simulink model "c00012M_harness"  (R2018a)
settings: Solver=FixedStepAuto  StartTime=0.0  StopTime=300  FixedStep=0.1  RelTol=1e-3
undefined symbols (not defined in the file): A1, hmax, PriorityTank, R1, R2, sigbuilder_block
(part 3 of 19)

== system c00012M_harness/Eval71 ==
  In1 : Inport
  In2 : Inport  Port=2
  Constant3 : Constant
  Data Type Conversion : DataTypeConversion
  Data Type Conversion1 : DataTypeConversion
  Memory1 : Memory  InitialCondition=1
  Memory2 : Memory  InitialCondition=1
  MinMax : MinMax  Inputs=3
  MinMax1 : MinMax  Inputs=2
  MinMax2 : MinMax  Inputs=2
  ROOut1 : RelationalOperator  Operator===  OutDataTypeStr=boolean  RndMeth=Simplest
  ROOut2 : RelationalOperator  Operator===  OutDataTypeStr=boolean  RndMeth=Simplest
  Out1 : Outport
  wires:
  Data Type Conversion1/1 -> MinMax2/1
  Data Type Conversion/1 -> MinMax1/1
  MinMax1/1 -> Memory1/1, MinMax/1
  MinMax2/1 -> MinMax/2, Memory2/1
  ROOut1/1 -> Data Type Conversion/1
  Memory2/1 -> MinMax2/2
  ROOut2/1 -> Data Type Conversion1/1
  Memory1/1 -> MinMax1/2
  [out2] -> ROOut2/2
  In1/1 -> ROOut1/1
  In2/1 -> ROOut2/1
  [out1] -> ROOut1/2
  MinMax/1 -> Out1/1
  Constant3/1 -> MinMax/3

== system c00012M_harness/Eval72 ==
  In1 : Inport
  In2 : Inport  Port=2
  Constant3 : Constant
  Data Type Conversion : DataTypeConversion
  Data Type Conversion1 : DataTypeConversion
  Memory1 : Memory  InitialCondition=1
  Memory2 : Memory  InitialCondition=1
  MinMax : MinMax  Inputs=3
  MinMax1 : MinMax  Inputs=2
  MinMax2 : MinMax  Inputs=2
  ROOut1 : RelationalOperator  Operator===  OutDataTypeStr=boolean  RndMeth=Simplest
  ROOut2 : RelationalOperator  Operator===  OutDataTypeStr=boolean  RndMeth=Simplest
  Out1 : Outport
  wires:
  Data Type Conversion1/1 -> MinMax2/1
  Data Type Conversion/1 -> MinMax1/1
  MinMax1/1 -> Memory1/1, MinMax/1
  MinMax2/1 -> MinMax/2, Memory2/1
  ROOut1/1 -> Data Type Conversion/1
  Memory2/1 -> MinMax2/2
  ROOut2/1 -> Data Type Conversion1/1
  Memory1/1 -> MinMax1/2
  [out2] -> ROOut2/2
  In1/1 -> ROOut1/1
  In2/1 -> ROOut2/1
  [out1] -> ROOut1/2
  MinMax/1 -> Out1/1
  Constant3/1 -> MinMax/3

== system c00012M_harness/Eval73 ==
  In1 : Inport
  In2 : Inport  Port=2
  Constant3 : Constant
  Data Type Conversion : DataTypeConversion
  Data Type Conversion1 : DataTypeConversion
  Memory1 : Memory  InitialCondition=1
  Memory2 : Memory  InitialCondition=1
  MinMax : MinMax  Inputs=3
  MinMax1 : MinMax  Inputs=2
  MinMax2 : MinMax  Inputs=2
  ROOut1 : RelationalOperator  Operator===  OutDataTypeStr=boolean  RndMeth=Simplest
  ROOut2 : RelationalOperator  Operator===  OutDataTypeStr=boolean  RndMeth=Simplest
  Out1 : Outport
  wires:
  Data Type Conversion1/1 -> MinMax2/1
  Data Type Conversion/1 -> MinMax1/1
  MinMax1/1 -> Memory1/1, MinMax/1
  MinMax2/1 -> MinMax/2, Memory2/1
  ROOut1/1 -> Data Type Conversion/1
  Memory2/1 -> MinMax2/2
  ROOut2/1 -> Data Type Conversion1/1
  Memory1/1 -> MinMax1/2
  [out2] -> ROOut2/2
  In1/1 -> ROOut1/1
  In2/1 -> ROOut2/1
  [out1] -> ROOut1/2
  MinMax/1 -> Out1/1
  Constant3/1 -> MinMax/3

== system c00012M_harness/Eval74 ==
  In1 : Inport
  In2 : Inport  Port=2
  Constant3 : Constant
  Data Type Conversion : DataTypeConversion
  Data Type Conversion1 : DataTypeConversion
  Memory1 : Memory  InitialCondition=1
  Memory2 : Memory  InitialCondition=1
  MinMax : MinMax  Inputs=3
  MinMax1 : MinMax  Inputs=2
  MinMax2 : MinMax  Inputs=2
  ROOut1 : RelationalOperator  Operator===  OutDataTypeStr=boolean  RndMeth=Simplest
  ROOut2 : RelationalOperator  Operator===  OutDataTypeStr=boolean  RndMeth=Simplest
  Out1 : Outport
  wires:
  Data Type Conversion1/1 -> MinMax2/1
  Data Type Conversion/1 -> MinMax1/1
  MinMax1/1 -> Memory1/1, MinMax/1
  MinMax2/1 -> MinMax/2, Memory2/1
  ROOut1/1 -> Data Type Conversion/1
  Memory2/1 -> MinMax2/2
  ROOut2/1 -> Data Type Conversion1/1
  Memory1/1 -> MinMax1/2
  [out2] -> ROOut2/2
  In1/1 -> ROOut1/1
  In2/1 -> ROOut2/1
  [out1] -> ROOut1/2
  MinMax/1 -> Out1/1
  Constant3/1 -> MinMax/3

== system c00012M_harness/Eval75 ==
  In1 : Inport
  In2 : Inport  Port=2
  Constant3 : Constant
  Data Type Conversion : DataTypeConversion
  Data Type Conversion1 : DataTypeConversion
  Memory1 : Memory  InitialCondition=1
  Memory2 : Memory  InitialCondition=1
  MinMax : MinMax  Inputs=3
  MinMax1 : MinMax  Inputs=2
  MinMax2 : MinMax  Inputs=2
  ROOut1 : RelationalOperator  Operator===  OutDataTypeStr=boolean  RndMeth=Simplest
  ROOut2 : RelationalOperator  Operator===  OutDataTypeStr=boolean  RndMeth=Simplest
  Out1 : Outport
  wires:
  Data Type Conversion1/1 -> MinMax2/1
  Data Type Conversion/1 -> MinMax1/1
  MinMax1/1 -> Memory1/1, MinMax/1
  MinMax2/1 -> MinMax/2, Memory2/1
  ROOut1/1 -> Data Type Conversion/1
  Memory2/1 -> MinMax2/2
  ROOut2/1 -> Data Type Conversion1/1
  Memory1/1 -> MinMax1/2
  [out2] -> ROOut2/2
  In1/1 -> ROOut1/1
  In2/1 -> ROOut2/1
  [out1] -> ROOut1/2
  MinMax/1 -> Out1/1
  Constant3/1 -> MinMax/3

== system c00012M_harness/Eval76 ==
  In1 : Inport
  In2 : Inport  Port=2
  Constant3 : Constant
  Data Type Conversion : DataTypeConversion
  Data Type Conversion1 : DataTypeConversion
  Memory1 : Memory  InitialCondition=1
  Memory2 : Memory  InitialCondition=1
  MinMax : MinMax  Inputs=3
  MinMax1 : MinMax  Inputs=2
  MinMax2 : MinMax  Inputs=2
  ROOut1 : RelationalOperator  Operator===  OutDataTypeStr=boolean  RndMeth=Simplest
  ROOut2 : RelationalOperator  Operator===  OutDataTypeStr=boolean  RndMeth=Simplest
  Out1 : Outport
  wires:
  Data Type Conversion1/1 -> MinMax2/1
  Data Type Conversion/1 -> MinMax1/1
  MinMax1/1 -> Memory1/1, MinMax/1
  MinMax2/1 -> MinMax/2, Memory2/1
  ROOut1/1 -> Data Type Conversion/1
  Memory2/1 -> MinMax2/2
  ROOut2/1 -> Data Type Conversion1/1
  Memory1/1 -> MinMax1/2
  [out2] -> ROOut2/2
  In1/1 -> ROOut1/1
  In2/1 -> ROOut2/1
  [out1] -> ROOut1/2
  MinMax/1 -> Out1/1
  Constant3/1 -> MinMax/3

== system c00012M_harness/Eval77 ==
  In1 : Inport
  In2 : Inport  Port=2
  Constant3 : Constant
  Data Type Conversion : DataTypeConversion
  Data Type Conversion1 : DataTypeConversion
  Memory1 : Memory  InitialCondition=1
  Memory2 : Memory  InitialCondition=1
  MinMax : MinMax  Inputs=3
  MinMax1 : MinMax  Inputs=2
  MinMax2 : MinMax  Inputs=2
  ROOut1 : RelationalOperator  Operator===  OutDataTypeStr=boolean  RndMeth=Simplest
  ROOut2 : RelationalOperator  Operator===  OutDataTypeStr=boolean  RndMeth=Simplest
  Out1 : Outport
  wires:
  Data Type Conversion1/1 -> MinMax2/1
  Data Type Conversion/1 -> MinMax1/1
  MinMax1/1 -> Memory1/1, MinMax/1
  MinMax2/1 -> MinMax/2, Memory2/1
  ROOut1/1 -> Data Type Conversion/1
  Memory2/1 -> MinMax2/2
  ROOut2/1 -> Data Type Conversion1/1
  Memory1/1 -> MinMax1/2
  [out2] -> ROOut2/2
  In1/1 -> ROOut1/1
  In2/1 -> ROOut2/1
  [out1] -> ROOut1/2
  MinMax/1 -> Out1/1
  Constant3/1 -> MinMax/3

== system c00012M_harness/Eval78 ==
  In1 : Inport
  In2 : Inport  Port=2
  Constant3 : Constant
  Data Type Conversion : DataTypeConversion
  Data Type Conversion1 : DataTypeConversion
  Memory1 : Memory  InitialCondition=1
  Memory2 : Memory  InitialCondition=1
  MinMax : MinMax  Inputs=3
  MinMax1 : MinMax  Inputs=2
  MinMax2 : MinMax  Inputs=2
  ROOut1 : RelationalOperator  Operator===  OutDataTypeStr=boolean  RndMeth=Simplest
  ROOut2 : RelationalOperator  Operator===  OutDataTypeStr=boolean  RndMeth=Simplest
  Out1 : Outport
  wires:
  Data Type Conversion1/1 -> MinMax2/1
  Data Type Conversion/1 -> MinMax1/1
  MinMax1/1 -> Memory1/1, MinMax/1
  MinMax2/1 -> MinMax/2, Memory2/1
  ROOut1/1 -> Data Type Conversion/1
  Memory2/1 -> MinMax2/2
  ROOut2/1 -> Data Type Conversion1/1
  Memory1/1 -> MinMax1/2
  [out2] -> ROOut2/2
  In1/1 -> ROOut1/1
  In2/1 -> ROOut2/1
  [out1] -> ROOut1/2
  MinMax/1 -> Out1/1
  Constant3/1 -> MinMax/3

== system c00012M_harness/Eval79 ==
  In1 : Inport
  In2 : Inport  Port=2
  Constant3 : Constant
  Data Type Conversion : DataTypeConversion
  Data Type Conversion1 : DataTypeConversion
  Memory1 : Memory  InitialCondition=1
  Memory2 : Memory  InitialCondition=1
  MinMax : MinMax  Inputs=3
  MinMax1 : MinMax  Inputs=2
  MinMax2 : MinMax  Inputs=2
  ROOut1 : RelationalOperator  Operator===  OutDataTypeStr=boolean  RndMeth=Simplest
  ROOut2 : RelationalOperator  Operator===  OutDataTypeStr=boolean  RndMeth=Simplest
  Out1 : Outport
  wires:
  Data Type Conversion1/1 -> MinMax2/1
  Data Type Conversion/1 -> MinMax1/1
  MinMax1/1 -> Memory1/1, MinMax/1
  MinMax2/1 -> MinMax/2, Memory2/1
  ROOut1/1 -> Data Type Conversion/1
  Memory2/1 -> MinMax2/2
  ROOut2/1 -> Data Type Conversion1/1
  Memory1/1 -> MinMax1/2
  [out2] -> ROOut2/2
  In1/1 -> ROOut1/1
  In2/1 -> ROOut2/1
  [out1] -> ROOut1/2
  MinMax/1 -> Out1/1
  Constant3/1 -> MinMax/3

== system c00012M_harness/Eval80 ==
  In1 : Inport
  In2 : Inport  Port=2
  Constant3 : Constant
  Data Type Conversion : DataTypeConversion
  Data Type Conversion1 : DataTypeConversion
  Memory1 : Memory  InitialCondition=1
  Memory2 : Memory  InitialCondition=1
  MinMax : MinMax  Inputs=3
  MinMax1 : MinMax  Inputs=2
  MinMax2 : MinMax  Inputs=2
  ROOut1 : RelationalOperator  Operator===  OutDataTypeStr=boolean  RndMeth=Simplest
  ROOut2 : RelationalOperator  Operator===  OutDataTypeStr=boolean  RndMeth=Simplest
  Out1 : Outport
  wires:
  Data Type Conversion1/1 -> MinMax2/1
  Data Type Conversion/1 -> MinMax1/1
  MinMax1/1 -> Memory1/1, MinMax/1
  MinMax2/1 -> MinMax/2, Memory2/1
  ROOut1/1 -> Data Type Conversion/1
  Memory2/1 -> MinMax2/2
  ROOut2/1 -> Data Type Conversion1/1
  Memory1/1 -> MinMax1/2
  [out2] -> ROOut2/2
  In1/1 -> ROOut1/1
  In2/1 -> ROOut2/1
  [out1] -> ROOut1/2
  MinMax/1 -> Out1/1
  Constant3/1 -> MinMax/3

== system c00012M_harness/Eval81 ==
  In1 : Inport
  In2 : Inport  Port=2
  Constant3 : Constant
  Data Type Conversion : DataTypeConversion
  Data Type Conversion1 : DataTypeConversion
  Memory1 : Memory  InitialCondition=1
  Memory2 : Memory  InitialCondition=1
  MinMax : MinMax  Inputs=3
  MinMax1 : MinMax  Inputs=2
  MinMax2 : MinMax  Inputs=2
  ROOut1 : RelationalOperator  Operator===  OutDataTypeStr=boolean  RndMeth=Simplest
  ROOut2 : RelationalOperator  Operator===  OutDataTypeStr=boolean  RndMeth=Simplest
  Out1 : Outport
  wires:
  Data Type Conversion1/1 -> MinMax2/1
  Data Type Conversion/1 -> MinMax1/1
  MinMax1/1 -> Memory1/1, MinMax/1
  MinMax2/1 -> MinMax/2, Memory2/1
  ROOut1/1 -> Data Type Conversion/1
  Memory2/1 -> MinMax2/2
  ROOut2/1 -> Data Type Conversion1/1
  Memory1/1 -> MinMax1/2
  [out2] -> ROOut2/2
  In1/1 -> ROOut1/1
  In2/1 -> ROOut2/1
  [out1] -> ROOut1/2
  MinMax/1 -> Out1/1
  Constant3/1 -> MinMax/3

== system c00012M_harness/Eval82 ==
  In1 : Inport
  In2 : Inport  Port=2
  Constant3 : Constant
  Data Type Conversion : DataTypeConversion
  Data Type Conversion1 : DataTypeConversion
  Memory1 : Memory  InitialCondition=1
  Memory2 : Memory  InitialCondition=1
  MinMax : MinMax  Inputs=3
  MinMax1 : MinMax  Inputs=2
  MinMax2 : MinMax  Inputs=2
  ROOut1 : RelationalOperator  Operator===  OutDataTypeStr=boolean  RndMeth=Simplest
  ROOut2 : RelationalOperator  Operator===  OutDataTypeStr=boolean  RndMeth=Simplest
  Out1 : Outport
  wires:
  Data Type Conversion1/1 -> MinMax2/1
  Data Type Conversion/1 -> MinMax1/1
  MinMax1/1 -> Memory1/1, MinMax/1
  MinMax2/1 -> MinMax/2, Memory2/1
  ROOut1/1 -> Data Type Conversion/1
  Memory2/1 -> MinMax2/2
  ROOut2/1 -> Data Type Conversion1/1
  Memory1/1 -> MinMax1/2
  [out2] -> ROOut2/2
  In1/1 -> ROOut1/1
  In2/1 -> ROOut2/1
  [out1] -> ROOut1/2
  MinMax/1 -> Out1/1
  Constant3/1 -> MinMax/3

== system c00012M_harness/Inputs ==
  Demux : Demux  Tag=STV Demux  Outputs=10
  FromWs : FromWorkspace  Tag=STV FromWs  VariableName=tuvar  SampleTime=0
  CT1 : Outport  Tag=STV Outport
  F1 : Outport  Tag=STV Outport  Port=2
  E1 : Outport  Tag=STV Outport  Port=3
  T1 : Outport  Tag=STV Outport  Port=4
  EB1 : Outport  Tag=STV Outport  Port=5
  CT2 : Outport  Tag=STV Outport  Port=6
  F2 : Outport  Tag=STV Outport  Port=7
  E2 : Outport  Tag=STV Outport  Port=8
  T2 : Outport  Tag=STV Outport  Port=9
  EB2 : Outport  Tag=STV Outport  Port=10
  wires:
  Demux/10 -> EB2/1
  Demux/9 -> T2/1
  Demux/8 -> E2/1
  Demux/7 -> F2/1
  Demux/6 -> CT2/1
  Demux/5 -> EB1/1
  Demux/4 -> T1/1
  Demux/3 -> E1/1
  Demux/2 -> F1/1
  Demux/1 -> CT1/1
  FromWs/1 -> Demux/1

== system c00012M_harness/M001 ==
  note: Inputs For Tank1
  note: Inputs For Tank3
  note: NAMES
      | --------------------------------------------
      | CT1 = ControlType Tank 1
      | F1 = Fill Tank 1
      | E1 = Empty Tank 1
      | MR1 = Manual Reference Tank1
      | T1 = Temperature Tank 1
      | EB1 = Emergency Button Tank 1
      | LL1 = Liquid Level 1
  note: Inputs For Tank2
  note: VALUES
      | ---------------------------------
      | ControlType = 1 | 2 | 3
      | FillTank = 0 | 1
      | EmptyTank = 0 | 1
      | ManualReference between 0 and 1
      | Tempreature between 0 and 100
      | EmergencyButton = 0 | 1
      | LiquidLevel between 0 and 1 (hmax)
  CT1 : Inport
  F1 : Inport  Port=2
  E1 : Inport  Port=3
  T1 : Inport  Port=4
  EB1 : Inport  Port=5
  CT2 : Inport  Port=6
  F2 : Inport  Port=7
  E2 : Inport  Port=8
  T2 : Inport  Port=9
  EB2 : Inport  Port=10
  Tank1 : Subsystem
  Tank2 : Subsystem
  LL1 : Outport
  LL2 : Outport  Port=2
  wires:
  CT1/1 -> Tank1/1(CT1)
  T2/1 -> Tank2/4(T2)
  E1/1 -> Tank1/3(E1)
  F1/1 -> Tank1/2(F1)
  E2/1 -> Tank2/3(E2)
  F2/1 -> Tank2/2(F2)
  Tank1/1(LL1) -> LL1/1, Tank2/6(LL1)
  T1/1 -> Tank1/4(T1)
  CT2/1 -> Tank2/1(CT2)
  EB2/1 -> Tank2/5(EB2)
  Tank2/1(LL2) -> LL2/1, Tank1/6(LL2)
  EB1/1 -> Tank1/5(EB1)

== system c00012M_harness/M036 ==
  note: VALUES
      | ---------------------------------
      | ControlType = 1 | 2 | 3
      | FillTank = 0 | 1
      | EmptyTank = 0 | 1
      | ManualReference between 0 and 1
      | Tempreature between 0 and 100
      | EmergencyButton = 0 | 1
      | LiquidLevel between 0 and 1 (hmax)
  note: Inputs For Tank2
  note: NAMES
      | --------------------------------------------
      | CT1 = ControlType Tank 1
      | F1 = Fill Tank 1
      | E1 = Empty Tank 1
      | MR1 = Manual Reference Tank1
      | T1 = Temperature Tank 1
      | EB1 = Emergency Button Tank 1
      | LL1 = Liquid Level 1
  note: Inputs For Tank3
  note: Inputs For Tank1
  CT1 : Inport
  F1 : Inport  Port=2
  E1 : Inport  Port=3
  T1 : Inport  Port=4
  EB1 : Inport  Port=5
  CT2 : Inport  Port=6
  F2 : Inport  Port=7
  E2 : Inport  Port=8
  T2 : Inport  Port=9
  EB2 : Inport  Port=10
  Tank1 : Subsystem
  Tank2 : Subsystem
  LL1 : Outport
  LL2 : Outport  Port=2
  wires:
  EB1/1 -> Tank1/5(EB1)
  Tank2/1(LL2) -> LL2/1, Tank1/6(LL2)
  EB2/1 -> Tank2/5(EB2)
  CT2/1 -> Tank2/1(CT2)
  T1/1 -> Tank1/4(T1)
  Tank1/1(LL1) -> LL1/1, Tank2/6(LL1)
  F2/1 -> Tank2/2(F2)
  E2/1 -> Tank2/3(E2)
  F1/1 -> Tank1/2(F1)
  E1/1 -> Tank1/3(E1)
  T2/1 -> Tank2/4(T2)
  CT1/1 -> Tank1/1(CT1)

== system c00012M_harness/M037 ==
  note: VALUES
      | ---------------------------------
      | ControlType = 1 | 2 | 3
      | FillTank = 0 | 1
      | EmptyTank = 0 | 1
      | ManualReference between 0 and 1
      | Tempreature between 0 and 100
      | EmergencyButton = 0 | 1
      | LiquidLevel between 0 and 1 (hmax)
  note: Inputs For Tank2
  note: NAMES
      | --------------------------------------------
      | CT1 = ControlType Tank 1
      | F1 = Fill Tank 1
      | E1 = Empty Tank 1
      | MR1 = Manual Reference Tank1
      | T1 = Temperature Tank 1
      | EB1 = Emergency Button Tank 1
      | LL1 = Liquid Level 1
  note: Inputs For Tank3
  note: Inputs For Tank1
  CT1 : Inport
  F1 : Inport  Port=2
  E1 : Inport  Port=3
  T1 : Inport  Port=4
  EB1 : Inport  Port=5
  CT2 : Inport  Port=6
  F2 : Inport  Port=7
  E2 : Inport  Port=8
  T2 : Inport  Port=9
  EB2 : Inport  Port=10
  Tank1 : Subsystem
  Tank2 : Subsystem
  LL1 : Outport
  LL2 : Outport  Port=2
  wires:
  EB1/1 -> Tank1/5(EB1)
  Tank2/1(LL2) -> LL2/1, Tank1/6(LL2)
  EB2/1 -> Tank2/5(EB2)
  CT2/1 -> Tank2/1(CT2)
  T1/1 -> Tank1/4(T1)
  Tank1/1(LL1) -> LL1/1, Tank2/6(LL1)
  F2/1 -> Tank2/2(F2)
  E2/1 -> Tank2/3(E2)
  F1/1 -> Tank1/2(F1)
  E1/1 -> Tank1/3(E1)
  T2/1 -> Tank2/4(T2)
  CT1/1 -> Tank1/1(CT1)

== system c00012M_harness/M038 ==
  note: VALUES
      | ---------------------------------
      | ControlType = 1 | 2 | 3
      | FillTank = 0 | 1
      | EmptyTank = 0 | 1
      | ManualReference between 0 and 1
      | Tempreature between 0 and 100
      | EmergencyButton = 0 | 1
      | LiquidLevel between 0 and 1 (hmax)
  note: Inputs For Tank2
  note: NAMES
      | --------------------------------------------
      | CT1 = ControlType Tank 1
      | F1 = Fill Tank 1
      | E1 = Empty Tank 1
      | MR1 = Manual Reference Tank1
      | T1 = Temperature Tank 1
      | EB1 = Emergency Button Tank 1
      | LL1 = Liquid Level 1
  note: Inputs For Tank3
  note: Inputs For Tank1
  CT1 : Inport
  F1 : Inport  Port=2
  E1 : Inport  Port=3
  T1 : Inport  Port=4
  EB1 : Inport  Port=5
  CT2 : Inport  Port=6
  F2 : Inport  Port=7
  E2 : Inport  Port=8
  T2 : Inport  Port=9
  EB2 : Inport  Port=10
  Tank1 : Subsystem
  Tank2 : Subsystem
  LL1 : Outport
  LL2 : Outport  Port=2
  wires:
  EB1/1 -> Tank1/5(EB1)
  Tank2/1(LL2) -> LL2/1, Tank1/6(LL2)
  EB2/1 -> Tank2/5(EB2)
  CT2/1 -> Tank2/1(CT2)
  T1/1 -> Tank1/4(T1)
  Tank1/1(LL1) -> LL1/1, Tank2/6(LL1)
  F2/1 -> Tank2/2(F2)
  E2/1 -> Tank2/3(E2)
  F1/1 -> Tank1/2(F1)
  E1/1 -> Tank1/3(E1)
  T2/1 -> Tank2/4(T2)
  CT1/1 -> Tank1/1(CT1)

== system c00012M_harness/M039 ==
  note: VALUES
      | ---------------------------------
      | ControlType = 1 | 2 | 3
      | FillTank = 0 | 1
      | EmptyTank = 0 | 1
      | ManualReference between 0 and 1
      | Tempreature between 0 and 100
      | EmergencyButton = 0 | 1
      | LiquidLevel between 0 and 1 (hmax)
  note: Inputs For Tank2
  note: NAMES
      | --------------------------------------------
      | CT1 = ControlType Tank 1
      | F1 = Fill Tank 1
      | E1 = Empty Tank 1
      | MR1 = Manual Reference Tank1
      | T1 = Temperature Tank 1
      | EB1 = Emergency Button Tank 1
      | LL1 = Liquid Level 1
  note: Inputs For Tank3
  note: Inputs For Tank1
  CT1 : Inport
  F1 : Inport  Port=2
  E1 : Inport  Port=3
  T1 : Inport  Port=4
  EB1 : Inport  Port=5
  CT2 : Inport  Port=6
  F2 : Inport  Port=7
  E2 : Inport  Port=8
  T2 : Inport  Port=9
  EB2 : Inport  Port=10
  Tank1 : Subsystem
  Tank2 : Subsystem
  LL1 : Outport
  LL2 : Outport  Port=2
  wires:
  EB1/1 -> Tank1/5(EB1)
  Tank2/1(LL2) -> LL2/1, Tank1/6(LL2)
  EB2/1 -> Tank2/5(EB2)
  CT2/1 -> Tank2/1(CT2)
  T1/1 -> Tank1/4(T1)
  Tank1/1(LL1) -> LL1/1, Tank2/6(LL1)
  F2/1 -> Tank2/2(F2)
  E2/1 -> Tank2/3(E2)
  F1/1 -> Tank1/2(F1)
  E1/1 -> Tank1/3(E1)
  T2/1 -> Tank2/4(T2)
  CT1/1 -> Tank1/1(CT1)

== system c00012M_harness/M040 ==
  note: VALUES
      | ---------------------------------
      | ControlType = 1 | 2 | 3
      | FillTank = 0 | 1
      | EmptyTank = 0 | 1
      | ManualReference between 0 and 1
      | Tempreature between 0 and 100
      | EmergencyButton = 0 | 1
      | LiquidLevel between 0 and 1 (hmax)
  note: Inputs For Tank2
  note: NAMES
      | --------------------------------------------
      | CT1 = ControlType Tank 1
      | F1 = Fill Tank 1
      | E1 = Empty Tank 1
      | MR1 = Manual Reference Tank1
      | T1 = Temperature Tank 1
      | EB1 = Emergency Button Tank 1
      | LL1 = Liquid Level 1
  note: Inputs For Tank3
  note: Inputs For Tank1
  CT1 : Inport
  F1 : Inport  Port=2
  E1 : Inport  Port=3
  T1 : Inport  Port=4
  EB1 : Inport  Port=5
  CT2 : Inport  Port=6
  F2 : Inport  Port=7
  E2 : Inport  Port=8
  T2 : Inport  Port=9
  EB2 : Inport  Port=10
  Tank1 : Subsystem
  Tank2 : Subsystem
  LL1 : Outport
  LL2 : Outport  Port=2
  wires:
  EB1/1 -> Tank1/5(EB1)
  Tank2/1(LL2) -> LL2/1, Tank1/6(LL2)
  EB2/1 -> Tank2/5(EB2)
  CT2/1 -> Tank2/1(CT2)
  T1/1 -> Tank1/4(T1)
  Tank1/1(LL1) -> LL1/1, Tank2/6(LL1)
  F2/1 -> Tank2/2(F2)
  E2/1 -> Tank2/3(E2)
  F1/1 -> Tank1/2(F1)
  E1/1 -> Tank1/3(E1)
  T2/1 -> Tank2/4(T2)
  CT1/1 -> Tank1/1(CT1)

== system c00012M_harness/M041 ==
  note: VALUES
      | ---------------------------------
      | ControlType = 1 | 2 | 3
      | FillTank = 0 | 1
      | EmptyTank = 0 | 1
      | ManualReference between 0 and 1
      | Tempreature between 0 and 100
      | EmergencyButton = 0 | 1
      | LiquidLevel between 0 and 1 (hmax)
  note: Inputs For Tank2
  note: NAMES
      | --------------------------------------------
      | CT1 = ControlType Tank 1
      | F1 = Fill Tank 1
      | E1 = Empty Tank 1
      | MR1 = Manual Reference Tank1
      | T1 = Temperature Tank 1
      | EB1 = Emergency Button Tank 1
      | LL1 = Liquid Level 1
  note: Inputs For Tank3
  note: Inputs For Tank1
  CT1 : Inport
  F1 : Inport  Port=2
  E1 : Inport  Port=3
  T1 : Inport  Port=4
  EB1 : Inport  Port=5
  CT2 : Inport  Port=6
  F2 : Inport  Port=7
  E2 : Inport  Port=8
  T2 : Inport  Port=9
  EB2 : Inport  Port=10
  Tank1 : Subsystem
  Tank2 : Subsystem
  LL1 : Outport
  LL2 : Outport  Port=2
  wires:
  EB1/1 -> Tank1/5(EB1)
  Tank2/1(LL2) -> LL2/1, Tank1/6(LL2)
  EB2/1 -> Tank2/5(EB2)
  CT2/1 -> Tank2/1(CT2)
  T1/1 -> Tank1/4(T1)
  Tank1/1(LL1) -> LL1/1, Tank2/6(LL1)
  F2/1 -> Tank2/2(F2)
  E2/1 -> Tank2/3(E2)
  F1/1 -> Tank1/2(F1)
  E1/1 -> Tank1/3(E1)
  T2/1 -> Tank2/4(T2)
  CT1/1 -> Tank1/1(CT1)

== system c00012M_harness/M042 ==
  note: VALUES
      | ---------------------------------
      | ControlType = 1 | 2 | 3
      | FillTank = 0 | 1
      | EmptyTank = 0 | 1
      | ManualReference between 0 and 1
      | Tempreature between 0 and 100
      | EmergencyButton = 0 | 1
      | LiquidLevel between 0 and 1 (hmax)
  note: Inputs For Tank2
  note: NAMES
      | --------------------------------------------
      | CT1 = ControlType Tank 1
      | F1 = Fill Tank 1
      | E1 = Empty Tank 1
      | MR1 = Manual Reference Tank1
      | T1 = Temperature Tank 1
      | EB1 = Emergency Button Tank 1
      | LL1 = Liquid Level 1
  note: Inputs For Tank3
  note: Inputs For Tank1
  CT1 : Inport
  F1 : Inport  Port=2
  E1 : Inport  Port=3
  T1 : Inport  Port=4
  EB1 : Inport  Port=5
  CT2 : Inport  Port=6
  F2 : Inport  Port=7
  E2 : Inport  Port=8
  T2 : Inport  Port=9
  EB2 : Inport  Port=10
  Tank1 : Subsystem
  Tank2 : Subsystem
  LL1 : Outport
  LL2 : Outport  Port=2
  wires:
  EB1/1 -> Tank1/5(EB1)
  Tank2/1(LL2) -> LL2/1, Tank1/6(LL2)
  EB2/1 -> Tank2/5(EB2)
  CT2/1 -> Tank2/1(CT2)
  T1/1 -> Tank1/4(T1)
  Tank1/1(LL1) -> LL1/1, Tank2/6(LL1)
  F2/1 -> Tank2/2(F2)
  E2/1 -> Tank2/3(E2)
  F1/1 -> Tank1/2(F1)
  E1/1 -> Tank1/3(E1)
  T2/1 -> Tank2/4(T2)
  CT1/1 -> Tank1/1(CT1)

== system c00012M_harness/M043 ==
  note: VALUES
      | ---------------------------------
      | ControlType = 1 | 2 | 3
      | FillTank = 0 | 1
      | EmptyTank = 0 | 1
      | ManualReference between 0 and 1
      | Tempreature between 0 and 100
      | EmergencyButton = 0 | 1
      | LiquidLevel between 0 and 1 (hmax)
  note: Inputs For Tank2
  note: NAMES
      | --------------------------------------------
      | CT1 = ControlType Tank 1
      | F1 = Fill Tank 1
      | E1 = Empty Tank 1
      | MR1 = Manual Reference Tank1
      | T1 = Temperature Tank 1
      | EB1 = Emergency Button Tank 1
      | LL1 = Liquid Level 1
  note: Inputs For Tank3
  note: Inputs For Tank1
  CT1 : Inport
  F1 : Inport  Port=2
  E1 : Inport  Port=3
  T1 : Inport  Port=4
  EB1 : Inport  Port=5
  CT2 : Inport  Port=6
  F2 : Inport  Port=7
  E2 : Inport  Port=8
  T2 : Inport  Port=9
  EB2 : Inport  Port=10
  Tank1 : Subsystem
  Tank2 : Subsystem
  LL1 : Outport
  LL2 : Outport  Port=2
  wires:
  EB1/1 -> Tank1/5(EB1)
  Tank2/1(LL2) -> LL2/1, Tank1/6(LL2)
  EB2/1 -> Tank2/5(EB2)
  CT2/1 -> Tank2/1(CT2)
  T1/1 -> Tank1/4(T1)
  Tank1/1(LL1) -> LL1/1, Tank2/6(LL1)
  F2/1 -> Tank2/2(F2)
  E2/1 -> Tank2/3(E2)
  F1/1 -> Tank1/2(F1)
  E1/1 -> Tank1/3(E1)
  T2/1 -> Tank2/4(T2)
  CT1/1 -> Tank1/1(CT1)

== system c00012M_harness/M044 ==
  note: VALUES
      | ---------------------------------
      | ControlType = 1 | 2 | 3
      | FillTank = 0 | 1
      | EmptyTank = 0 | 1
      | ManualReference between 0 and 1
      | Tempreature between 0 and 100
      | EmergencyButton = 0 | 1
      | LiquidLevel between 0 and 1 (hmax)
  note: Inputs For Tank2
  note: NAMES
      | --------------------------------------------
      | CT1 = ControlType Tank 1
      | F1 = Fill Tank 1
      | E1 = Empty Tank 1
      | MR1 = Manual Reference Tank1
      | T1 = Temperature Tank 1
      | EB1 = Emergency Button Tank 1
      | LL1 = Liquid Level 1
  note: Inputs For Tank3
  note: Inputs For Tank1
  CT1 : Inport
  F1 : Inport  Port=2
  E1 : Inport  Port=3
  T1 : Inport  Port=4
  EB1 : Inport  Port=5
  CT2 : Inport  Port=6
  F2 : Inport  Port=7
  E2 : Inport  Port=8
  T2 : Inport  Port=9
  EB2 : Inport  Port=10
  Tank1 : Subsystem
  Tank2 : Subsystem
  LL1 : Outport
  LL2 : Outport  Port=2
  wires:
  EB1/1 -> Tank1/5(EB1)
  Tank2/1(LL2) -> LL2/1, Tank1/6(LL2)
  EB2/1 -> Tank2/5(EB2)
  CT2/1 -> Tank2/1(CT2)
  T1/1 -> Tank1/4(T1)
  Tank1/1(LL1) -> LL1/1, Tank2/6(LL1)
  F2/1 -> Tank2/2(F2)
  E2/1 -> Tank2/3(E2)
  F1/1 -> Tank1/2(F1)
  E1/1 -> Tank1/3(E1)
  T2/1 -> Tank2/4(T2)
  CT1/1 -> Tank1/1(CT1)

== system c00012M_harness/M045 ==
  note: VALUES
      | ---------------------------------
      | ControlType = 1 | 2 | 3
      | FillTank = 0 | 1
      | EmptyTank = 0 | 1
      | ManualReference between 0 and 1
      | Tempreature between 0 and 100
      | EmergencyButton = 0 | 1
      | LiquidLevel between 0 and 1 (hmax)
  note: Inputs For Tank2
  note: NAMES
      | --------------------------------------------
      | CT1 = ControlType Tank 1
      | F1 = Fill Tank 1
      | E1 = Empty Tank 1
      | MR1 = Manual Reference Tank1
      | T1 = Temperature Tank 1
      | EB1 = Emergency Button Tank 1
      | LL1 = Liquid Level 1
  note: Inputs For Tank3
  note: Inputs For Tank1
  CT1 : Inport
  F1 : Inport  Port=2
  E1 : Inport  Port=3
  T1 : Inport  Port=4
  EB1 : Inport  Port=5
  CT2 : Inport  Port=6
  F2 : Inport  Port=7
  E2 : Inport  Port=8
  T2 : Inport  Port=9
  EB2 : Inport  Port=10
  Tank1 : Subsystem
  Tank2 : Subsystem
  LL1 : Outport
  LL2 : Outport  Port=2
  wires:
  EB1/1 -> Tank1/5(EB1)
  Tank2/1(LL2) -> LL2/1, Tank1/6(LL2)
  EB2/1 -> Tank2/5(EB2)
  CT2/1 -> Tank2/1(CT2)
  T1/1 -> Tank1/4(T1)
  Tank1/1(LL1) -> LL1/1, Tank2/6(LL1)
  F2/1 -> Tank2/2(F2)
  E2/1 -> Tank2/3(E2)
  F1/1 -> Tank1/2(F1)
  E1/1 -> Tank1/3(E1)
  T2/1 -> Tank2/4(T2)
  CT1/1 -> Tank1/1(CT1)

== system c00012M_harness/M058 ==
  note: VALUES
      | ---------------------------------
      | ControlType = 1 | 2 | 3
      | FillTank = 0 | 1
      | EmptyTank = 0 | 1
      | ManualReference between 0 and 1
      | Tempreature between 0 and 100
      | EmergencyButton = 0 | 1
      | LiquidLevel between 0 and 1 (hmax)
  note: Inputs For Tank2
  note: NAMES
      | --------------------------------------------
      | CT1 = ControlType Tank 1
      | F1 = Fill Tank 1
      | E1 = Empty Tank 1
      | MR1 = Manual Reference Tank1
      | T1 = Temperature Tank 1
      | EB1 = Emergency Button Tank 1
      | LL1 = Liquid Level 1
  note: Inputs For Tank3
  note: Inputs For Tank1
  CT1 : Inport
  F1 : Inport  Port=2
  E1 : Inport  Port=3
  T1 : Inport  Port=4
  EB1 : Inport  Port=5
  CT2 : Inport  Port=6
  F2 : Inport  Port=7
  E2 : Inport  Port=8
  T2 : Inport  Port=9
  EB2 : Inport  Port=10
  Tank1 : Subsystem
  Tank2 : Subsystem
  LL1 : Outport
  LL2 : Outport  Port=2
  wires:
  EB1/1 -> Tank1/5(EB1)
  Tank2/1(LL2) -> LL2/1, Tank1/6(LL2)
  EB2/1 -> Tank2/5(EB2)
  CT2/1 -> Tank2/1(CT2)
  T1/1 -> Tank1/4(T1)
  Tank1/1(LL1) -> LL1/1, Tank2/6(LL1)
  F2/1 -> Tank2/2(F2)
  E2/1 -> Tank2/3(E2)
  F1/1 -> Tank1/2(F1)
  E1/1 -> Tank1/3(E1)
  T2/1 -> Tank2/4(T2)
  CT1/1 -> Tank1/1(CT1)

== system c00012M_harness/M059 ==
  note: VALUES
      | ---------------------------------
      | ControlType = 1 | 2 | 3
      | FillTank = 0 | 1
      | EmptyTank = 0 | 1
      | ManualReference between 0 and 1
      | Tempreature between 0 and 100
      | EmergencyButton = 0 | 1
      | LiquidLevel between 0 and 1 (hmax)
  note: Inputs For Tank2
  note: NAMES
      | --------------------------------------------
      | CT1 = ControlType Tank 1
      | F1 = Fill Tank 1
      | E1 = Empty Tank 1
      | MR1 = Manual Reference Tank1
      | T1 = Temperature Tank 1
      | EB1 = Emergency Button Tank 1
      | LL1 = Liquid Level 1
  note: Inputs For Tank3
  note: Inputs For Tank1
  CT1 : Inport
  F1 : Inport  Port=2
  E1 : Inport  Port=3
  T1 : Inport  Port=4
  EB1 : Inport  Port=5
  CT2 : Inport  Port=6
  F2 : Inport  Port=7
  E2 : Inport  Port=8
  T2 : Inport  Port=9
  EB2 : Inport  Port=10
  Tank1 : Subsystem
  Tank2 : Subsystem
  LL1 : Outport
  LL2 : Outport  Port=2
  wires:
  EB1/1 -> Tank1/5(EB1)
  Tank2/1(LL2) -> LL2/1, Tank1/6(LL2)
  EB2/1 -> Tank2/5(EB2)
  CT2/1 -> Tank2/1(CT2)
  T1/1 -> Tank1/4(T1)
  Tank1/1(LL1) -> LL1/1, Tank2/6(LL1)
  F2/1 -> Tank2/2(F2)
  E2/1 -> Tank2/3(E2)
  F1/1 -> Tank1/2(F1)
  E1/1 -> Tank1/3(E1)
  T2/1 -> Tank2/4(T2)
  CT1/1 -> Tank1/1(CT1)

== system c00012M_harness/M060 ==
  note: VALUES
      | ---------------------------------
      | ControlType = 1 | 2 | 3
      | FillTank = 0 | 1
      | EmptyTank = 0 | 1
      | ManualReference between 0 and 1
      | Tempreature between 0 and 100
      | EmergencyButton = 0 | 1
      | LiquidLevel between 0 and 1 (hmax)
  note: Inputs For Tank2
  note: NAMES
      | --------------------------------------------
      | CT1 = ControlType Tank 1
      | F1 = Fill Tank 1
      | E1 = Empty Tank 1
      | MR1 = Manual Reference Tank1
      | T1 = Temperature Tank 1
      | EB1 = Emergency Button Tank 1
      | LL1 = Liquid Level 1
  note: Inputs For Tank3
  note: Inputs For Tank1
  CT1 : Inport
  F1 : Inport  Port=2
  E1 : Inport  Port=3
  T1 : Inport  Port=4
  EB1 : Inport  Port=5
  CT2 : Inport  Port=6
  F2 : Inport  Port=7
  E2 : Inport  Port=8
  T2 : Inport  Port=9
  EB2 : Inport  Port=10
  Tank1 : Subsystem
  Tank2 : Subsystem
  LL1 : Outport
  LL2 : Outport  Port=2
  wires:
  EB1/1 -> Tank1/5(EB1)
  Tank2/1(LL2) -> LL2/1, Tank1/6(LL2)
  EB2/1 -> Tank2/5(EB2)
  CT2/1 -> Tank2/1(CT2)
  T1/1 -> Tank1/4(T1)
  Tank1/1(LL1) -> LL1/1, Tank2/6(LL1)
  F2/1 -> Tank2/2(F2)
  E2/1 -> Tank2/3(E2)
  F1/1 -> Tank1/2(F1)
  E1/1 -> Tank1/3(E1)
  T2/1 -> Tank2/4(T2)
  CT1/1 -> Tank1/1(CT1)

== system c00012M_harness/M061 ==
  note: VALUES
      | ---------------------------------
      | ControlType = 1 | 2 | 3
      | FillTank = 0 | 1
      | EmptyTank = 0 | 1
      | ManualReference between 0 and 1
      | Tempreature between 0 and 100
      | EmergencyButton = 0 | 1
      | LiquidLevel between 0 and 1 (hmax)
  note: Inputs For Tank2
  note: NAMES
      | --------------------------------------------
      | CT1 = ControlType Tank 1
      | F1 = Fill Tank 1
      | E1 = Empty Tank 1
      | MR1 = Manual Reference Tank1
      | T1 = Temperature Tank 1
      | EB1 = Emergency Button Tank 1
      | LL1 = Liquid Level 1
  note: Inputs For Tank3
  note: Inputs For Tank1
  CT1 : Inport
  F1 : Inport  Port=2
  E1 : Inport  Port=3
  T1 : Inport  Port=4
  EB1 : Inport  Port=5
  CT2 : Inport  Port=6
  F2 : Inport  Port=7
  E2 : Inport  Port=8
  T2 : Inport  Port=9
  EB2 : Inport  Port=10
  Tank1 : Subsystem
  Tank2 : Subsystem
  LL1 : Outport
  LL2 : Outport  Port=2
  wires:
  EB1/1 -> Tank1/5(EB1)
  Tank2/1(LL2) -> LL2/1, Tank1/6(LL2)
  EB2/1 -> Tank2/5(EB2)
  CT2/1 -> Tank2/1(CT2)
  T1/1 -> Tank1/4(T1)
  Tank1/1(LL1) -> LL1/1, Tank2/6(LL1)
  F2/1 -> Tank2/2(F2)
  E2/1 -> Tank2/3(E2)
  F1/1 -> Tank1/2(F1)
  E1/1 -> Tank1/3(E1)
  T2/1 -> Tank2/4(T2)
  CT1/1 -> Tank1/1(CT1)

== system c00012M_harness/M062 ==
  note: VALUES
      | ---------------------------------
      | ControlType = 1 | 2 | 3
      | FillTank = 0 | 1
      | EmptyTank = 0 | 1
      | ManualReference between 0 and 1
      | Tempreature between 0 and 100
      | EmergencyButton = 0 | 1
      | LiquidLevel between 0 and 1 (hmax)
  note: Inputs For Tank2
  note: NAMES
      | --------------------------------------------
      | CT1 = ControlType Tank 1
      | F1 = Fill Tank 1
      | E1 = Empty Tank 1
      | MR1 = Manual Reference Tank1
      | T1 = Temperature Tank 1
      | EB1 = Emergency Button Tank 1
      | LL1 = Liquid Level 1
  note: Inputs For Tank3
  note: Inputs For Tank1
  CT1 : Inport
  F1 : Inport  Port=2
  E1 : Inport  Port=3
  T1 : Inport  Port=4
  EB1 : Inport  Port=5
  CT2 : Inport  Port=6
  F2 : Inport  Port=7
  E2 : Inport  Port=8
  T2 : Inport  Port=9
  EB2 : Inport  Port=10
  Tank1 : Subsystem
  Tank2 : Subsystem
  LL1 : Outport
  LL2 : Outport  Port=2
  wires:
  EB1/1 -> Tank1/5(EB1)
  Tank2/1(LL2) -> LL2/1, Tank1/6(LL2)
  EB2/1 -> Tank2/5(EB2)
  CT2/1 -> Tank2/1(CT2)
  T1/1 -> Tank1/4(T1)
  Tank1/1(LL1) -> LL1/1, Tank2/6(LL1)
  F2/1 -> Tank2/2(F2)
  E2/1 -> Tank2/3(E2)
  F1/1 -> Tank1/2(F1)
  E1/1 -> Tank1/3(E1)
  T2/1 -> Tank2/4(T2)
  CT1/1 -> Tank1/1(CT1)

== system c00012M_harness/M063 ==
  note: VALUES
      | ---------------------------------
      | ControlType = 1 | 2 | 3
      | FillTank = 0 | 1
      | EmptyTank = 0 | 1
      | ManualReference between 0 and 1
      | Tempreature between 0 and 100
      | EmergencyButton = 0 | 1
      | LiquidLevel between 0 and 1 (hmax)
  note: Inputs For Tank2
  note: NAMES
      | --------------------------------------------
      | CT1 = ControlType Tank 1
      | F1 = Fill Tank 1
      | E1 = Empty Tank 1
      | MR1 = Manual Reference Tank1
      | T1 = Temperature Tank 1
      | EB1 = Emergency Button Tank 1
      | LL1 = Liquid Level 1
  note: Inputs For Tank3
  note: Inputs For Tank1
  CT1 : Inport
  F1 : Inport  Port=2
  E1 : Inport  Port=3
  T1 : Inport  Port=4
  EB1 : Inport  Port=5
  CT2 : Inport  Port=6
  F2 : Inport  Port=7
  E2 : Inport  Port=8
  T2 : Inport  Port=9
  EB2 : Inport  Port=10
  Tank1 : Subsystem
  Tank2 : Subsystem
  LL1 : Outport
  LL2 : Outport  Port=2
  wires:
  EB1/1 -> Tank1/5(EB1)
  Tank2/1(LL2) -> LL2/1, Tank1/6(LL2)
  EB2/1 -> Tank2/5(EB2)
  CT2/1 -> Tank2/1(CT2)
  T1/1 -> Tank1/4(T1)
  Tank1/1(LL1) -> LL1/1, Tank2/6(LL1)
  F2/1 -> Tank2/2(F2)
  E2/1 -> Tank2/3(E2)
  F1/1 -> Tank1/2(F1)
  E1/1 -> Tank1/3(E1)
  T2/1 -> Tank2/4(T2)
  CT1/1 -> Tank1/1(CT1)

== system c00012M_harness/M064 ==
  note: VALUES
      | ---------------------------------
      | ControlType = 1 | 2 | 3
      | FillTank = 0 | 1
      | EmptyTank = 0 | 1
      | ManualReference between 0 and 1
      | Tempreature between 0 and 100
      | EmergencyButton = 0 | 1
      | LiquidLevel between 0 and 1 (hmax)
  note: Inputs For Tank2
  note: NAMES
      | --------------------------------------------
      | CT1 = ControlType Tank 1
      | F1 = Fill Tank 1
      | E1 = Empty Tank 1
      | MR1 = Manual Reference Tank1
      | T1 = Temperature Tank 1
      | EB1 = Emergency Button Tank 1
      | LL1 = Liquid Level 1
  note: Inputs For Tank3
  note: Inputs For Tank1
  CT1 : Inport
  F1 : Inport  Port=2
  E1 : Inport  Port=3
  T1 : Inport  Port=4
  EB1 : Inport  Port=5
  CT2 : Inport  Port=6
  F2 : Inport  Port=7
  E2 : Inport  Port=8
  T2 : Inport  Port=9
  EB2 : Inport  Port=10
  Tank1 : Subsystem
  Tank2 : Subsystem
  LL1 : Outport
  LL2 : Outport  Port=2
  wires:
  EB1/1 -> Tank1/5(EB1)
  Tank2/1(LL2) -> LL2/1, Tank1/6(LL2)
  EB2/1 -> Tank2/5(EB2)
  CT2/1 -> Tank2/1(CT2)
  T1/1 -> Tank1/4(T1)
  Tank1/1(LL1) -> LL1/1, Tank2/6(LL1)
  F2/1 -> Tank2/2(F2)
  E2/1 -> Tank2/3(E2)
  F1/1 -> Tank1/2(F1)
  E1/1 -> Tank1/3(E1)
  T2/1 -> Tank2/4(T2)
  CT1/1 -> Tank1/1(CT1)

== system c00012M_harness/M065 ==
  note: VALUES
      | ---------------------------------
      | ControlType = 1 | 2 | 3
      | FillTank = 0 | 1
      | EmptyTank = 0 | 1
      | ManualReference between 0 and 1
      | Tempreature between 0 and 100
      | EmergencyButton = 0 | 1
      | LiquidLevel between 0 and 1 (hmax)
  note: Inputs For Tank2
  note: NAMES
      | --------------------------------------------
      | CT1 = ControlType Tank 1
      | F1 = Fill Tank 1
      | E1 = Empty Tank 1
      | MR1 = Manual Reference Tank1
      | T1 = Temperature Tank 1
      | EB1 = Emergency Button Tank 1
      | LL1 = Liquid Level 1
  note: Inputs For Tank3
  note: Inputs For Tank1
  CT1 : Inport
  F1 : Inport  Port=2
  E1 : Inport  Port=3
  T1 : Inport  Port=4
  EB1 : Inport  Port=5
  CT2 : Inport  Port=6
  F2 : Inport  Port=7
  E2 : Inport  Port=8
  T2 : Inport  Port=9
  EB2 : Inport  Port=10
  Tank1 : Subsystem
  Tank2 : Subsystem
  LL1 : Outport
  LL2 : Outport  Port=2
  wires:
  EB1/1 -> Tank1/5(EB1)
  Tank2/1(LL2) -> LL2/1, Tank1/6(LL2)
  EB2/1 -> Tank2/5(EB2)
  CT2/1 -> Tank2/1(CT2)
  T1/1 -> Tank1/4(T1)
  Tank1/1(LL1) -> LL1/1, Tank2/6(LL1)
  F2/1 -> Tank2/2(F2)
  E2/1 -> Tank2/3(E2)
  F1/1 -> Tank1/2(F1)
  E1/1 -> Tank1/3(E1)
  T2/1 -> Tank2/4(T2)
  CT1/1 -> Tank1/1(CT1)

== system c00012M_harness/M066 ==
  note: VALUES
      | ---------------------------------
      | ControlType = 1 | 2 | 3
      | FillTank = 0 | 1
      | EmptyTank = 0 | 1
      | ManualReference between 0 and 1
      | Tempreature between 0 and 100
      | EmergencyButton = 0 | 1
      | LiquidLevel between 0 and 1 (hmax)
  note: Inputs For Tank2
  note: NAMES
      | --------------------------------------------
      | CT1 = ControlType Tank 1
      | F1 = Fill Tank 1
      | E1 = Empty Tank 1
      | MR1 = Manual Reference Tank1
      | T1 = Temperature Tank 1
      | EB1 = Emergency Button Tank 1
      | LL1 = Liquid Level 1
  note: Inputs For Tank3
  note: Inputs For Tank1
  CT1 : Inport
  F1 : Inport  Port=2
  E1 : Inport  Port=3
  T1 : Inport  Port=4
  EB1 : Inport  Port=5
  CT2 : Inport  Port=6
  F2 : Inport  Port=7
  E2 : Inport  Port=8
  T2 : Inport  Port=9
  EB2 : Inport  Port=10
  Tank1 : Subsystem
  Tank2 : Subsystem
  LL1 : Outport
  LL2 : Outport  Port=2
  wires:
  EB1/1 -> Tank1/5(EB1)
  Tank2/1(LL2) -> LL2/1, Tank1/6(LL2)
  EB2/1 -> Tank2/5(EB2)
  CT2/1 -> Tank2/1(CT2)
  T1/1 -> Tank1/4(T1)
  Tank1/1(LL1) -> LL1/1, Tank2/6(LL1)
  F2/1 -> Tank2/2(F2)
  E2/1 -> Tank2/3(E2)
  F1/1 -> Tank1/2(F1)
  E1/1 -> Tank1/3(E1)
  T2/1 -> Tank2/4(T2)
  CT1/1 -> Tank1/1(CT1)

== system c00012M_harness/M067 ==
  note: VALUES
      | ---------------------------------
      | ControlType = 1 | 2 | 3
      | FillTank = 0 | 1
      | EmptyTank = 0 | 1
      | ManualReference between 0 and 1
      | Tempreature between 0 and 100
      | EmergencyButton = 0 | 1
      | LiquidLevel between 0 and 1 (hmax)
  note: Inputs For Tank2
  note: NAMES
      | --------------------------------------------
      | CT1 = ControlType Tank 1
      | F1 = Fill Tank 1
      | E1 = Empty Tank 1
      | MR1 = Manual Reference Tank1
      | T1 = Temperature Tank 1
      | EB1 = Emergency Button Tank 1
      | LL1 = Liquid Level 1
  note: Inputs For Tank3
  note: Inputs For Tank1
  CT1 : Inport
  F1 : Inport  Port=2
  E1 : Inport  Port=3
  T1 : Inport  Port=4
  EB1 : Inport  Port=5
  CT2 : Inport  Port=6
  F2 : Inport  Port=7
  E2 : Inport  Port=8
  T2 : Inport  Port=9
  EB2 : Inport  Port=10
  Tank1 : Subsystem
  Tank2 : Subsystem
  LL1 : Outport
  LL2 : Outport  Port=2
  wires:
  EB1/1 -> Tank1/5(EB1)
  Tank2/1(LL2) -> LL2/1, Tank1/6(LL2)
  EB2/1 -> Tank2/5(EB2)
  CT2/1 -> Tank2/1(CT2)
  T1/1 -> Tank1/4(T1)
  Tank1/1(LL1) -> LL1/1, Tank2/6(LL1)
  F2/1 -> Tank2/2(F2)
  E2/1 -> Tank2/3(E2)
  F1/1 -> Tank1/2(F1)
  E1/1 -> Tank1/3(E1)
  T2/1 -> Tank2/4(T2)
  CT1/1 -> Tank1/1(CT1)

== system c00012M_harness/M068 ==
  note: VALUES
      | ---------------------------------
      | ControlType = 1 | 2 | 3
      | FillTank = 0 | 1
      | EmptyTank = 0 | 1
      | ManualReference between 0 and 1
      | Tempreature between 0 and 100
      | EmergencyButton = 0 | 1
      | LiquidLevel between 0 and 1 (hmax)
  note: Inputs For Tank2
  note: NAMES
      | --------------------------------------------
      | CT1 = ControlType Tank 1
      | F1 = Fill Tank 1
      | E1 = Empty Tank 1
      | MR1 = Manual Reference Tank1
      | T1 = Temperature Tank 1
      | EB1 = Emergency Button Tank 1
      | LL1 = Liquid Level 1
  note: Inputs For Tank3
  note: Inputs For Tank1
  CT1 : Inport
  F1 : Inport  Port=2
  E1 : Inport  Port=3
  T1 : Inport  Port=4
  EB1 : Inport  Port=5
  CT2 : Inport  Port=6
  F2 : Inport  Port=7
  E2 : Inport  Port=8
  T2 : Inport  Port=9
  EB2 : Inport  Port=10
  Tank1 : Subsystem
  Tank2 : Subsystem
  LL1 : Outport
  LL2 : Outport  Port=2
  wires:
  EB1/1 -> Tank1/5(EB1)
  Tank2/1(LL2) -> LL2/1, Tank1/6(LL2)
  EB2/1 -> Tank2/5(EB2)
  CT2/1 -> Tank2/1(CT2)
  T1/1 -> Tank1/4(T1)
  Tank1/1(LL1) -> LL1/1, Tank2/6(LL1)
  F2/1 -> Tank2/2(F2)
  E2/1 -> Tank2/3(E2)
  F1/1 -> Tank1/2(F1)
  E1/1 -> Tank1/3(E1)
  T2/1 -> Tank2/4(T2)
  CT1/1 -> Tank1/1(CT1)

== system c00012M_harness/M069 ==
  note: VALUES
      | ---------------------------------
      | ControlType = 1 | 2 | 3
      | FillTank = 0 | 1
      | EmptyTank = 0 | 1
      | ManualReference between 0 and 1
      | Tempreature between 0 and 100
      | EmergencyButton = 0 | 1
      | LiquidLevel between 0 and 1 (hmax)
  note: Inputs For Tank2
  note: NAMES
      | --------------------------------------------
      | CT1 = ControlType Tank 1
      | F1 = Fill Tank 1
      | E1 = Empty Tank 1
      | MR1 = Manual Reference Tank1
      | T1 = Temperature Tank 1
      | EB1 = Emergency Button Tank 1
      | LL1 = Liquid Level 1
  note: Inputs For Tank3
  note: Inputs For Tank1
  CT1 : Inport
  F1 : Inport  Port=2
  E1 : Inport  Port=3
  T1 : Inport  Port=4
  EB1 : Inport  Port=5
  CT2 : Inport  Port=6
  F2 : Inport  Port=7
  E2 : Inport  Port=8
  T2 : Inport  Port=9
  EB2 : Inport  Port=10
  Tank1 : Subsystem
  Tank2 : Subsystem
  LL1 : Outport
  LL2 : Outport  Port=2
  wires:
  EB1/1 -> Tank1/5(EB1)
  Tank2/1(LL2) -> LL2/1, Tank1/6(LL2)
  EB2/1 -> Tank2/5(EB2)
  CT2/1 -> Tank2/1(CT2)
  T1/1 -> Tank1/4(T1)
  Tank1/1(LL1) -> LL1/1, Tank2/6(LL1)
  F2/1 -> Tank2/2(F2)
  E2/1 -> Tank2/3(E2)
  F1/1 -> Tank1/2(F1)
  E1/1 -> Tank1/3(E1)
  T2/1 -> Tank2/4(T2)
  CT1/1 -> Tank1/1(CT1)

== system c00012M_harness/M070 ==
  note: VALUES
      | ---------------------------------
      | ControlType = 1 | 2 | 3
      | FillTank = 0 | 1
      | EmptyTank = 0 | 1
      | ManualReference between 0 and 1
      | Tempreature between 0 and 100
      | EmergencyButton = 0 | 1
      | LiquidLevel between 0 and 1 (hmax)
  note: Inputs For Tank2
  note: NAMES
      | --------------------------------------------
      | CT1 = ControlType Tank 1
      | F1 = Fill Tank 1
      | E1 = Empty Tank 1
      | MR1 = Manual Reference Tank1
      | T1 = Temperature Tank 1
      | EB1 = Emergency Button Tank 1
      | LL1 = Liquid Level 1
  note: Inputs For Tank3
  note: Inputs For Tank1
  CT1 : Inport
  F1 : Inport  Port=2
  E1 : Inport  Port=3
  T1 : Inport  Port=4
  EB1 : Inport  Port=5
  CT2 : Inport  Port=6
  F2 : Inport  Port=7
  E2 : Inport  Port=8
  T2 : Inport  Port=9
  EB2 : Inport  Port=10
  Tank1 : Subsystem
  Tank2 : Subsystem
  LL1 : Outport
  LL2 : Outport  Port=2
  wires:
  EB1/1 -> Tank1/5(EB1)
  Tank2/1(LL2) -> LL2/1, Tank1/6(LL2)
  EB2/1 -> Tank2/5(EB2)
  CT2/1 -> Tank2/1(CT2)
  T1/1 -> Tank1/4(T1)
  Tank1/1(LL1) -> LL1/1, Tank2/6(LL1)
  F2/1 -> Tank2/2(F2)
  E2/1 -> Tank2/3(E2)
  F1/1 -> Tank1/2(F1)
  E1/1 -> Tank1/3(E1)
  T2/1 -> Tank2/4(T2)
  CT1/1 -> Tank1/1(CT1)

== system c00012M_harness/M071 ==
  note: VALUES
      | ---------------------------------
      | ControlType = 1 | 2 | 3
      | FillTank = 0 | 1
      | EmptyTank = 0 | 1
      | ManualReference between 0 and 1
      | Tempreature between 0 and 100
      | EmergencyButton = 0 | 1
      | LiquidLevel between 0 and 1 (hmax)
  note: Inputs For Tank2
  note: NAMES
      | --------------------------------------------
      | CT1 = ControlType Tank 1
      | F1 = Fill Tank 1
      | E1 = Empty Tank 1
      | MR1 = Manual Reference Tank1
      | T1 = Temperature Tank 1
      | EB1 = Emergency Button Tank 1
      | LL1 = Liquid Level 1
  note: Inputs For Tank3
  note: Inputs For Tank1
  CT1 : Inport
  F1 : Inport  Port=2
  E1 : Inport  Port=3
  T1 : Inport  Port=4
  EB1 : Inport  Port=5
  CT2 : Inport  Port=6
  F2 : Inport  Port=7
  E2 : Inport  Port=8
  T2 : Inport  Port=9
  EB2 : Inport  Port=10
  Tank1 : Subsystem
  Tank2 : Subsystem
  LL1 : Outport
  LL2 : Outport  Port=2
  wires:
  EB1/1 -> Tank1/5(EB1)
  Tank2/1(LL2) -> LL2/1, Tank1/6(LL2)
  EB2/1 -> Tank2/5(EB2)
  CT2/1 -> Tank2/1(CT2)
  T1/1 -> Tank1/4(T1)
  Tank1/1(LL1) -> LL1/1, Tank2/6(LL1)
  F2/1 -> Tank2/2(F2)
  E2/1 -> Tank2/3(E2)
  F1/1 -> Tank1/2(F1)
  E1/1 -> Tank1/3(E1)
  T2/1 -> Tank2/4(T2)
  CT1/1 -> Tank1/1(CT1)

== system c00012M_harness/M072 ==
  note: VALUES
      | ---------------------------------
      | ControlType = 1 | 2 | 3
      | FillTank = 0 | 1
      | EmptyTank = 0 | 1
      | ManualReference between 0 and 1
      | Tempreature between 0 and 100
      | EmergencyButton = 0 | 1
      | LiquidLevel between 0 and 1 (hmax)
  note: Inputs For Tank2
  note: NAMES
      | --------------------------------------------
      | CT1 = ControlType Tank 1
      | F1 = Fill Tank 1
      | E1 = Empty Tank 1
      | MR1 = Manual Reference Tank1
      | T1 = Temperature Tank 1
      | EB1 = Emergency Button Tank 1
      | LL1 = Liquid Level 1
  note: Inputs For Tank3
  note: Inputs For Tank1
  CT1 : Inport
  F1 : Inport  Port=2
  E1 : Inport  Port=3
  T1 : Inport  Port=4
  EB1 : Inport  Port=5
  CT2 : Inport  Port=6
  F2 : Inport  Port=7
  E2 : Inport  Port=8
  T2 : Inport  Port=9
  EB2 : Inport  Port=10
  Tank1 : Subsystem
  Tank2 : Subsystem
  LL1 : Outport
  LL2 : Outport  Port=2
  wires:
  EB1/1 -> Tank1/5(EB1)
  Tank2/1(LL2) -> LL2/1, Tank1/6(LL2)
  EB2/1 -> Tank2/5(EB2)
  CT2/1 -> Tank2/1(CT2)
  T1/1 -> Tank1/4(T1)
  Tank1/1(LL1) -> LL1/1, Tank2/6(LL1)
  F2/1 -> Tank2/2(F2)
  E2/1 -> Tank2/3(E2)
  F1/1 -> Tank1/2(F1)
  E1/1 -> Tank1/3(E1)
  T2/1 -> Tank2/4(T2)
  CT1/1 -> Tank1/1(CT1)

== system c00012M_harness/M073 ==
  note: VALUES
      | ---------------------------------
      | ControlType = 1 | 2 | 3
      | FillTank = 0 | 1
      | EmptyTank = 0 | 1
      | ManualReference between 0 and 1
      | Tempreature between 0 and 100
      | EmergencyButton = 0 | 1
      | LiquidLevel between 0 and 1 (hmax)
  note: Inputs For Tank2
  note: NAMES
      | --------------------------------------------
      | CT1 = ControlType Tank 1
      | F1 = Fill Tank 1
      | E1 = Empty Tank 1
      | MR1 = Manual Reference Tank1
      | T1 = Temperature Tank 1
      | EB1 = Emergency Button Tank 1
      | LL1 = Liquid Level 1
  note: Inputs For Tank3
  note: Inputs For Tank1
  CT1 : Inport
  F1 : Inport  Port=2
  E1 : Inport  Port=3
  T1 : Inport  Port=4
  EB1 : Inport  Port=5
  CT2 : Inport  Port=6
  F2 : Inport  Port=7
  E2 : Inport  Port=8
  T2 : Inport  Port=9
  EB2 : Inport  Port=10
  Tank1 : Subsystem
  Tank2 : Subsystem
  LL1 : Outport
  LL2 : Outport  Port=2
  wires:
  EB1/1 -> Tank1/5(EB1)
  Tank2/1(LL2) -> LL2/1, Tank1/6(LL2)
  EB2/1 -> Tank2/5(EB2)
  CT2/1 -> Tank2/1(CT2)
  T1/1 -> Tank1/4(T1)
  Tank1/1(LL1) -> LL1/1, Tank2/6(LL1)
  F2/1 -> Tank2/2(F2)
  E2/1 -> Tank2/3(E2)
  F1/1 -> Tank1/2(F1)
  E1/1 -> Tank1/3(E1)
  T2/1 -> Tank2/4(T2)
  CT1/1 -> Tank1/1(CT1)

== system c00012M_harness/M074 ==
  note: VALUES
      | ---------------------------------
      | ControlType = 1 | 2 | 3
      | FillTank = 0 | 1
      | EmptyTank = 0 | 1
      | ManualReference between 0 and 1
      | Tempreature between 0 and 100
      | EmergencyButton = 0 | 1
      | LiquidLevel between 0 and 1 (hmax)
  note: Inputs For Tank2
  note: NAMES
      | --------------------------------------------
      | CT1 = ControlType Tank 1
      | F1 = Fill Tank 1
      | E1 = Empty Tank 1
      | MR1 = Manual Reference Tank1
      | T1 = Temperature Tank 1
      | EB1 = Emergency Button Tank 1
      | LL1 = Liquid Level 1
  note: Inputs For Tank3
  note: Inputs For Tank1
  CT1 : Inport
  F1 : Inport  Port=2
  E1 : Inport  Port=3
  T1 : Inport  Port=4
  EB1 : Inport  Port=5
  CT2 : Inport  Port=6
  F2 : Inport  Port=7
  E2 : Inport  Port=8
  T2 : Inport  Port=9
  EB2 : Inport  Port=10
  Tank1 : Subsystem
  Tank2 : Subsystem
  LL1 : Outport
  LL2 : Outport  Port=2
  wires:
  EB1/1 -> Tank1/5(EB1)
  Tank2/1(LL2) -> LL2/1, Tank1/6(LL2)
  EB2/1 -> Tank2/5(EB2)
  CT2/1 -> Tank2/1(CT2)
  T1/1 -> Tank1/4(T1)
  Tank1/1(LL1) -> LL1/1, Tank2/6(LL1)
  F2/1 -> Tank2/2(F2)
  E2/1 -> Tank2/3(E2)
  F1/1 -> Tank1/2(F1)
  E1/1 -> Tank1/3(E1)
  T2/1 -> Tank2/4(T2)
  CT1/1 -> Tank1/1(CT1)

== system c00012M_harness/M075 ==
  note: VALUES
      | ---------------------------------
      | ControlType = 1 | 2 | 3
      | FillTank = 0 | 1
      | EmptyTank = 0 | 1
      | ManualReference between 0 and 1
      | Tempreature between 0 and 100
      | EmergencyButton = 0 | 1
      | LiquidLevel between 0 and 1 (hmax)
  note: Inputs For Tank2
  note: NAMES
      | --------------------------------------------
      | CT1 = ControlType Tank 1
      | F1 = Fill Tank 1
      | E1 = Empty Tank 1
      | MR1 = Manual Reference Tank1
      | T1 = Temperature Tank 1
      | EB1 = Emergency Button Tank 1
      | LL1 = Liquid Level 1
  note: Inputs For Tank3
  note: Inputs For Tank1
  CT1 : Inport
  F1 : Inport  Port=2
  E1 : Inport  Port=3
  T1 : Inport  Port=4
  EB1 : Inport  Port=5
  CT2 : Inport  Port=6
  F2 : Inport  Port=7
  E2 : Inport  Port=8
  T2 : Inport  Port=9
  EB2 : Inport  Port=10
  Tank1 : Subsystem
  Tank2 : Subsystem
  LL1 : Outport
  LL2 : Outport  Port=2
  wires:
  EB1/1 -> Tank1/5(EB1)
  Tank2/1(LL2) -> LL2/1, Tank1/6(LL2)
  EB2/1 -> Tank2/5(EB2)
  CT2/1 -> Tank2/1(CT2)
  T1/1 -> Tank1/4(T1)
  Tank1/1(LL1) -> LL1/1, Tank2/6(LL1)
  F2/1 -> Tank2/2(F2)
  E2/1 -> Tank2/3(E2)
  F1/1 -> Tank1/2(F1)
  E1/1 -> Tank1/3(E1)
  T2/1 -> Tank2/4(T2)
  CT1/1 -> Tank1/1(CT1)

== system c00012M_harness/M076 ==
  note: VALUES
      | ---------------------------------
      | ControlType = 1 | 2 | 3
      | FillTank = 0 | 1
      | EmptyTank = 0 | 1
      | ManualReference between 0 and 1
      | Tempreature between 0 and 100
      | EmergencyButton = 0 | 1
      | LiquidLevel between 0 and 1 (hmax)
  note: Inputs For Tank2
  note: NAMES
      | --------------------------------------------
      | CT1 = ControlType Tank 1
      | F1 = Fill Tank 1
      | E1 = Empty Tank 1
      | MR1 = Manual Reference Tank1
      | T1 = Temperature Tank 1
      | EB1 = Emergency Button Tank 1
      | LL1 = Liquid Level 1
  note: Inputs For Tank3
  note: Inputs For Tank1
  CT1 : Inport
  F1 : Inport  Port=2
  E1 : Inport  Port=3
  T1 : Inport  Port=4
  EB1 : Inport  Port=5
  CT2 : Inport  Port=6
  F2 : Inport  Port=7
  E2 : Inport  Port=8
  T2 : Inport  Port=9
  EB2 : Inport  Port=10
  Tank1 : Subsystem
  Tank2 : Subsystem
  LL1 : Outport
  LL2 : Outport  Port=2
  wires:
  EB1/1 -> Tank1/5(EB1)
  Tank2/1(LL2) -> LL2/1, Tank1/6(LL2)
  EB2/1 -> Tank2/5(EB2)
  CT2/1 -> Tank2/1(CT2)
  T1/1 -> Tank1/4(T1)
  Tank1/1(LL1) -> LL1/1, Tank2/6(LL1)
  F2/1 -> Tank2/2(F2)
  E2/1 -> Tank2/3(E2)
  F1/1 -> Tank1/2(F1)
  E1/1 -> Tank1/3(E1)
  T2/1 -> Tank2/4(T2)
  CT1/1 -> Tank1/1(CT1)

== system c00012M_harness/M077 ==
  note: VALUES
      | ---------------------------------
      | ControlType = 1 | 2 | 3
      | FillTank = 0 | 1
      | EmptyTank = 0 | 1
      | ManualReference between 0 and 1
      | Tempreature between 0 and 100
      | EmergencyButton = 0 | 1
      | LiquidLevel between 0 and 1 (hmax)
  note: Inputs For Tank2
  note: NAMES
      | --------------------------------------------
      | CT1 = ControlType Tank 1
      | F1 = Fill Tank 1
      | E1 = Empty Tank 1
      | MR1 = Manual Reference Tank1
      | T1 = Temperature Tank 1
      | EB1 = Emergency Button Tank 1
      | LL1 = Liquid Level 1
  note: Inputs For Tank3
  note: Inputs For Tank1
  CT1 : Inport
  F1 : Inport  Port=2
  E1 : Inport  Port=3
  T1 : Inport  Port=4
  EB1 : Inport  Port=5
  CT2 : Inport  Port=6
  F2 : Inport  Port=7
  E2 : Inport  Port=8
  T2 : Inport  Port=9
  EB2 : Inport  Port=10
  Tank1 : Subsystem
  Tank2 : Subsystem
  LL1 : Outport
  LL2 : Outport  Port=2
  wires:
  EB1/1 -> Tank1/5(EB1)
  Tank2/1(LL2) -> LL2/1, Tank1/6(LL2)
  EB2/1 -> Tank2/5(EB2)
  CT2/1 -> Tank2/1(CT2)
  T1/1 -> Tank1/4(T1)
  Tank1/1(LL1) -> LL1/1, Tank2/6(LL1)
  F2/1 -> Tank2/2(F2)
  E2/1 -> Tank2/3(E2)
  F1/1 -> Tank1/2(F1)
  E1/1 -> Tank1/3(E1)
  T2/1 -> Tank2/4(T2)
  CT1/1 -> Tank1/1(CT1)

== system c00012M_harness/M078 ==
  note: VALUES
      | ---------------------------------
      | ControlType = 1 | 2 | 3
      | FillTank = 0 | 1
      | EmptyTank = 0 | 1
      | ManualReference between 0 and 1
      | Tempreature between 0 and 100
      | EmergencyButton = 0 | 1
      | LiquidLevel between 0 and 1 (hmax)
  note: Inputs For Tank2
  note: NAMES
      | --------------------------------------------
      | CT1 = ControlType Tank 1
      | F1 = Fill Tank 1
      | E1 = Empty Tank 1
      | MR1 = Manual Reference Tank1
      | T1 = Temperature Tank 1
      | EB1 = Emergency Button Tank 1
      | LL1 = Liquid Level 1
  note: Inputs For Tank3
  note: Inputs For Tank1
  CT1 : Inport
  F1 : Inport  Port=2
  E1 : Inport  Port=3
  T1 : Inport  Port=4
  EB1 : Inport  Port=5
  CT2 : Inport  Port=6
  F2 : Inport  Port=7
  E2 : Inport  Port=8
  T2 : Inport  Port=9
  EB2 : Inport  Port=10
  Tank1 : Subsystem
  Tank2 : Subsystem
  LL1 : Outport
  LL2 : Outport  Port=2
  wires:
  EB1/1 -> Tank1/5(EB1)
  Tank2/1(LL2) -> LL2/1, Tank1/6(LL2)
  EB2/1 -> Tank2/5(EB2)
  CT2/1 -> Tank2/1(CT2)
  T1/1 -> Tank1/4(T1)
  Tank1/1(LL1) -> LL1/1, Tank2/6(LL1)
  F2/1 -> Tank2/2(F2)
  E2/1 -> Tank2/3(E2)
  F1/1 -> Tank1/2(F1)
  E1/1 -> Tank1/3(E1)
  T2/1 -> Tank2/4(T2)
  CT1/1 -> Tank1/1(CT1)
